simulink model "umpc_wl_qp_beckymod2"  (R2017a)
settings: Solver=FixedStepDiscrete  StartTime=0.0  StopTime=20  FixedStep=0.0002  RelTol=1e-3  EnableMultiTasking=on
values from neighbouring files (symbols this model uses):
  f_fin = f    (= 160)    [target_driver_setup.m]
  f_int = f    (= 160)    [target_driver_setup.m]
  kquad = [4e1, 1e-4, 4e-5, 153, 1e0]    [target_driver_setup.m]
  lpfParams = [0.2, 0.5, 1e-1, 1e1]    [target_driver_setup.m]
  phase = 0.0    (= 0)    [target_driver_setup.m]
  pos0 = [0.05,-0.02,0.08]    [target_driver_setup.m]
  running_time = 0.0+T+0.0    (= 2)    [target_driver_setup.m]
  start_delay = 0.0    (= 0)    [target_driver_setup.m]
  T = 2    [target_driver_setup.m]
  trajAmp = 0.07    [target_driver_setup.m]
  trajFreq = 0.5    [target_driver_setup.m]
  wmpc = single([3e2, 5e1, 1e-4, 2e-4, 1e0, 1e0, 1e-1, 1e0])    [target_driver_setup.m]
undefined symbols (not defined in the file or in its folder): Com1, DiscIntNeverNeededParam, none
libraries: simulink x9, xpcnilib x2, xpcseriallib x2, xpcutilitieslib x1

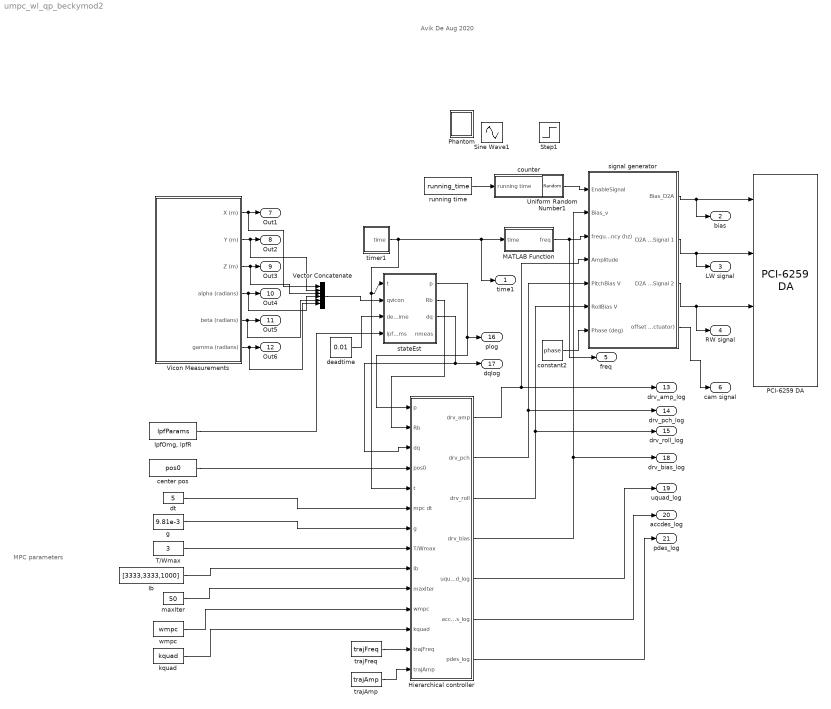
== system umpc_wl_qp_beckymod2 ==
  note: Avik De
      | Aug 2020
  note: MPC parameters
  Hierarchical controller : Subsystem
  Ib : Constant  Value=[3333,3333,1000]  OutDataTypeStr=single  SampleTime=-1
  MATLAB Function : MATLAB Function  TreatAsAtomicUnit=on
  PCI-6259 DA : xpcnilib/D//A/M Series/PCI-6259 DA  channel=[1:4]  range=[10,5, 10, 10]  reset=[1 1 1 1]  initValue=[0 0 0 0]  sampletime=-1  slot=-1
  Phantom : Subsystem
  T/Wmax : Constant  Value=3  OutDataTypeStr=single  SampleTime=-1
  Vector Concatenate : Concatenate  NumInputs=6
  Vicon Measurements : Subsystem
  center pos : Constant  Value=pos0  OutDataTypeStr=single  SampleTime=-1
  constant2 : Constant  Value=phase
  counter : Subsystem
  deadtime : Constant  Value=0.01
  dt : Constant  Value=5  OutDataTypeStr=single  SampleTime=-1
  g : Constant  Value=9.81e-3  OutDataTypeStr=single  SampleTime=-1
  kquad : Constant  Value=kquad  VectorParams1D=off  OutDataTypeStr=single  SampleTime=-1
  "lpfOmg, lpfR" : Constant  Value=lpfParams  VectorParams1D=off  OutDataTypeStr=double  SampleTime=-1
  maxIter : Constant  Value=50  OutDataTypeStr=int32  SampleTime=-1
  running time : Constant  Value=running_time  SampleTime=-1
  signal generator : Subsystem
  stateEst : MATLAB Function  TreatAsAtomicUnit=on
  timer1 : Subsystem
  trajAmp : Constant  Value=trajAmp  OutDataTypeStr=single  SampleTime=-1
  trajFreq : Constant  Value=trajFreq  OutDataTypeStr=single  SampleTime=-1
  wmpc : Constant  Value=wmpc  VectorParams1D=off  OutDataTypeStr=single  SampleTime=-1
  time1 : Outport
  bias : Outport  Port=2
  LW signal : Outport  Port=3
  RW signal : Outport  Port=4
  freq : Outport  Port=5
  cam signal : Outport  Port=6
  Out1 : Outport  Port=7
  Out2 : Outport  Port=8
  Out3 : Outport  Port=9
  Out4 : Outport  Port=10
  Out5 : Outport  Port=11
  Out6 : Outport  Port=12
  drv_amp_log : Outport  Port=13
  drv_pch_log : Outport  Port=14
  drv_roll_log : Outport  Port=15
  plog : Outport  Port=16
  dqlog : Outport  Port=17
  drv_bias_log : Outport  Port=18
  uquad_log : Outport  Port=19
  accdes_log : Outport  Port=20
  pdes_log : Outport  Port=21
  Sine Wave1 : Sin  IOType=siggen  SampleTime=0
  Step1 : Step  IOType=siggen  SampleTime=0
  Uniform Random Number1 : UniformRandomNumber  IOType=siggen  SampleTime=0
  wires:
  running time/1 -> counter/1(running time)
  signal generator/1(Bias_D2A) -> bias/1, PCI-6259 DA/1
  signal generator/2(D2A DriveSignal 1) -> LW signal/1, PCI-6259 DA/2
  signal generator/3(D2A DriveSignal 2) -> RW signal/1, PCI-6259 DA/3
  timer1/1(time) -> Hierarchical controller/5(t), stateEst/1(t), time1/1, MATLAB Function/1(time)
  counter/1(enable) -> signal generator/1(EnableSignal)
  MATLAB Function/1(freq) -> signal generator/3(frequency (hz)), freq/1
  signal generator/4(offset (for sylvain's actuator)) -> cam signal/1
  constant2/1 -> signal generator/7(Phase (deg))
  Vicon Measurements/1(X (m)) -> Vector Concatenate/1, Out1/1
  Vicon Measurements/6(gamma (radians)) -> Vector Concatenate/6, Out6/1
  Vicon Measurements/3(Z (m)) -> Vector Concatenate/3, Out3/1
  Vicon Measurements/2(Y (m)) -> Vector Concatenate/2, Out2/1
  Vicon Measurements/5(beta (radians)) -> Vector Concatenate/5, Out5/1
  Vicon Measurements/4(alpha (radians)) -> Vector Concatenate/4, Out4/1
  Hierarchical controller/1(drv_amp) -> drv_amp_log/1, signal generator/4(Amplitude)
  Hierarchical controller/3(drv_roll) -> signal generator/6(RollBias V), drv_roll_log/1
  Hierarchical controller/2(drv_pch) -> signal generator/5(PitchBias V), drv_pch_log/1
  stateEst/1(p) -> Hierarchical controller/1(p), plog/1
  stateEst/2(Rb) -> Hierarchical controller/2(Rb)
  stateEst/3(dq) -> dqlog/1, Hierarchical controller/3(dq)
  Vector Concatenate/1 -> stateEst/2(qvicon)
  Hierarchical controller/4(drv_bias) -> signal generator/2(Bias_v), drv_bias_log/1
  center pos/1 -> Hierarchical controller/4(pos0)
  dt/1 -> Hierarchical controller/6(mpc dt)
  g/1 -> Hierarchical controller/7(g)
  T/Wmax/1 -> Hierarchical controller/8(T/Wmax)
  wmpc/1 -> Hierarchical controller/11(wmpc)
  maxIter/1 -> Hierarchical controller/10(maxIter)
  Ib/1 -> Hierarchical controller/9(Ib)
  Hierarchical controller/5(uquad_log) -> uquad_log/1
  Hierarchical controller/6(accdes_log) -> accdes_log/1
  deadtime/1 -> stateEst/3(deadtime)
  kquad/1 -> Hierarchical controller/12(kquad)
  "lpfOmg, lpfR"/1 -> stateEst/4(lpfParams)
  Hierarchical controller/7(pdes_log) -> pdes_log/1
  trajFreq/1 -> Hierarchical controller/13(trajFreq)
  trajAmp/1 -> Hierarchical controller/14(trajAmp)

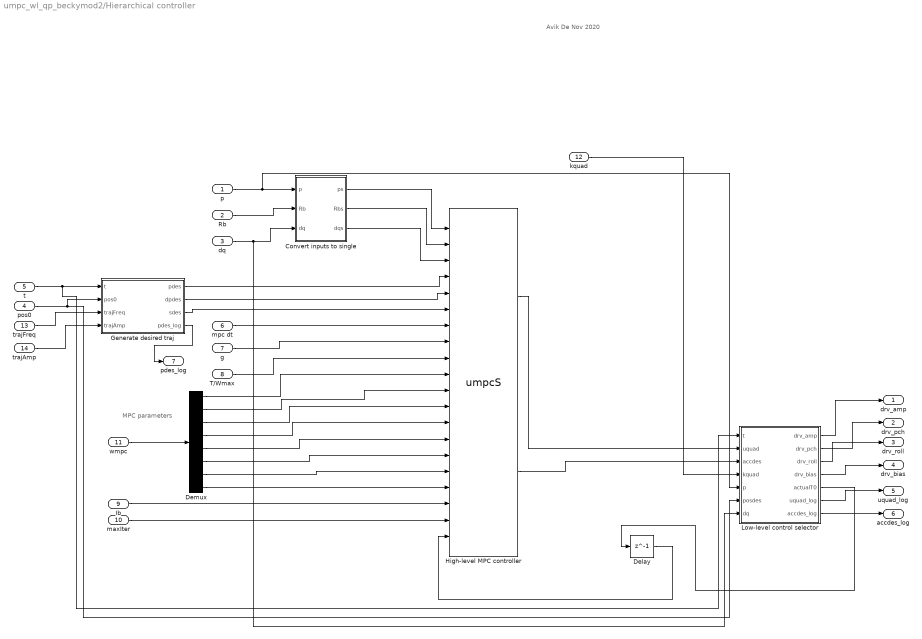
== system umpc_wl_qp_beckymod2/Hierarchical controller ==
  note: Avik De
      | Nov 2020
  note: MPC parameters
  p : Inport
  Rb : Inport  Port=2
  dq : Inport  Port=3
  pos0 : Inport  Port=4
  t : Inport  Port=5
  mpc dt : Inport  Port=6
  g : Inport  Port=7
  T/Wmax : Inport  Port=8
  Ib : Inport  Port=9
  maxIter : Inport  Port=10
  wmpc : Inport  Port=11
  kquad : Inport  Port=12
  trajFreq : Inport  Port=13
  trajAmp : Inport  Port=14
  Convert inputs to single : MATLAB Function  TreatAsAtomicUnit=on
  Delay : Delay  DelayLength=1  InitialCondition=0
  Demux : Demux  Outputs=8
  Generate desired traj : MATLAB Function  TreatAsAtomicUnit=on
  High-level MPC controller : S-Function  FunctionName=umpcS  Parameters=SampleTime  SFunctionDeploymentMode=off  EnableBusSupport=off  mask(Legacy Function){SFunctionSpec=void umpcS(single y1[3], single y2[6], single u1[3], single u2[3][3], single u3[6], single u4[3], single u5[3], single u6[3], single u7, single u8, single u9, single u10, single u11, single u12, single u13, single u14, single u15, single u16, single u17, single u18[3], int32 u19, single u20), SampleTime=-1, ShowSpec=off}
      mask prompts: SampleTime "Sample time (-1 for inherited):"; ShowSpec "Display function specification"
      mask help: This block allows you to call the legacy functions specified by the following Legacy Code Tool definition: def.SFunctionName = 'umpcS'; def.OutputFcnSpec = 'void umpcS(single y1[3], single y2[6], single u1[3], single u2[3][3], single u3[6], single u4[3], single u5[3], single u6[3], single u7, single u8, single u9, single u10, single u11, single u12, single u13, single u14, single u15, single u16, single u17, single u18[3], int32 u19, single u20)'; def.HeaderFiles = {'uprightmpc2.h'}; def.SourceFiles = {'uprightmpc2.c', 'eigenc.c', 'auxil.c', 'error.c', 'kkt.c', 'lin_alg.c', 'osqp.c', 'proj.c',
  Low-level control selector : MATLAB Function  TreatAsAtomicUnit=on
  drv_amp : Outport
  drv_pch : Outport  Port=2
  drv_roll : Outport  Port=3
  drv_bias : Outport  Port=4
  uquad_log : Outport  Port=5
  accdes_log : Outport  Port=6
  pdes_log : Outport  Port=7  OutDataTypeStr=double
  wires:
  Low-level control selector/2(drv_pch) -> drv_pch/1
  Low-level control selector/3(drv_roll) -> drv_roll/1
  Low-level control selector/4(drv_bias) -> drv_bias/1
  Low-level control selector/1(drv_amp) -> drv_amp/1
  pos0/1 -> Low-level control selector/6(posdes), Generate desired traj/2(pos0)
  mpc dt/1 -> High-level MPC controller/7
  g/1 -> High-level MPC controller/8
  T/Wmax/1 -> High-level MPC controller/9
  Demux/1 -> High-level MPC controller/10
  Demux/2 -> High-level MPC controller/11
  Demux/3 -> High-level MPC controller/12
  Demux/4 -> High-level MPC controller/13
  Demux/5 -> High-level MPC controller/14
  Demux/6 -> High-level MPC controller/15
  Demux/7 -> High-level MPC controller/16
  Demux/8 -> High-level MPC controller/17
  Ib/1 -> High-level MPC controller/18
  maxIter/1 -> High-level MPC controller/19
  High-level MPC controller/1 -> Low-level control selector/2(uquad)
  t/1 -> Low-level control selector/1(t), Generate desired traj/1(t)
  Generate desired traj/1(pdes) -> High-level MPC controller/4
  Generate desired traj/2(dpdes) -> High-level MPC controller/5
  Convert inputs to single/1(ps) -> High-level MPC controller/1
  Convert inputs to single/2(Rbs) -> High-level MPC controller/2
  Convert inputs to single/3(dqs) -> High-level MPC controller/3
  p/1 -> Low-level control selector/5(p), Convert inputs to single/1(p)
  Rb/1 -> Convert inputs to single/2(Rb)
  dq/1 -> Low-level control selector/7(dq), Convert inputs to single/3(dq)
  High-level MPC controller/2 -> Low-level control selector/3(accdes)
  Generate desired traj/3(sdes) -> High-level MPC controller/6
  Low-level control selector/6(uquad_log) -> uquad_log/1
  Low-level control selector/7(accdes_log) -> accdes_log/1
  Low-level control selector/5(actualT0) -> Delay/1
  Delay/1 -> High-level MPC controller/20
  wmpc/1 -> Demux/1
  kquad/1 -> Low-level control selector/4(kquad)
  trajFreq/1 -> Generate desired traj/3(trajFreq)
  trajAmp/1 -> Generate desired traj/4(trajAmp)
  Generate desired traj/4(pdes_log) -> pdes_log/1

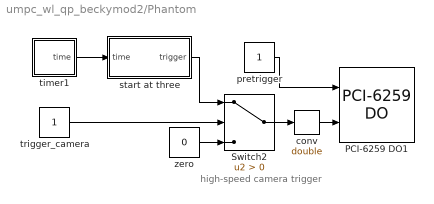
== system umpc_wl_qp_beckymod2/Phantom ==
  note: high-speed camera trigger
  PCI-6259 DO1 : xpcnilib/Digital Output/M Series/PCI-6259 DO  channel=[1 2]  reset=[0 0]  initValue=[0 0]  sampletime=0.0002  slot=-1
  Switch2 : Switch  Criteria=u2 > Threshold
  conv : DataTypeConversion  OutDataTypeStr=double
  pretrigger : Constant
  start at three : MATLAB Function  TreatAsAtomicUnit=on
  timer1 : Subsystem
  trigger_camera : Constant
  zero : Constant  Value=0
  wires:
  timer1/1(time) -> start at three/1(time)
  start at three/1(trigger) -> Switch2/1
  Switch2/1 -> conv/1
  zero/1 -> Switch2/3
  trigger_camera/1 -> Switch2/2
  conv/1 -> PCI-6259 DO1/2
  pretrigger/1 -> PCI-6259 DO1/1

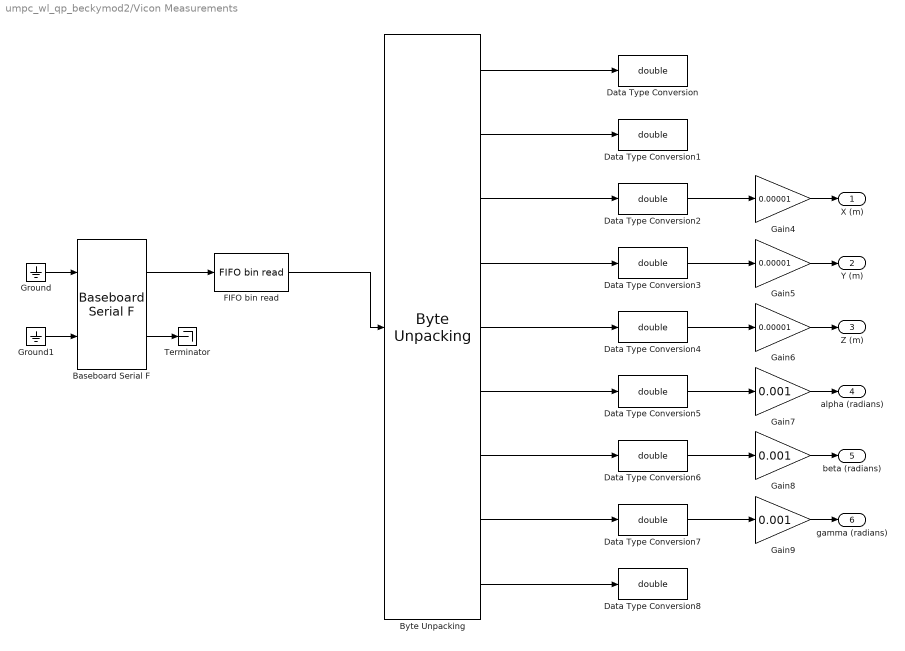
== system umpc_wl_qp_beckymod2/Vicon Measurements ==
  Baseboard Serial F : xpcseriallib/Mainboard/Baseboard Serial F  group=FIFO Setup  port=1  irqnum=4  saddr1=0x3f8  saddr2=0x3e8  config=Com1/none  baud1=115200  parity1=None  ndata1=8  nstop1=1  fifomode1=16 deep  rlevel1=half full  automode1=on  xmtfifosize1=1024  xmtdatatype1=8 bit int null terminated  rcvfifosize1=1024  baud2=115200  parity2=None  ndata2=8  nstop2=1  fifomode2=16 deep  rlevel2=half full  automode2=off  xmtfifosize2=1024  xmtdatatype2=8 bit uint null terminated  rcvfifosize2=1024
  "Byte Unpacking " : xpcutilitieslib/Byte Unpacking   MaskUnpackedDataTypes={'uint8','int16','int16','int16','int16','int16','int16','int16','uint8'}  MaskUnpackedDataSizes={[1] [1] [1] [1] [1] [1] [1] [1] [1]}  MaskAlignment=1
  Data Type Conversion{,1..8} (9 alike) : DataTypeConversion  OutDataTypeStr=double
  "FIFO bin read " : xpcseriallib/FIFO bin read   header=[128,127,127]  lengths=[15]  hold=Hold last output if no new data  enable=off  maxsize=15  outputtype=8 bit uint null terminated  sampletime=0.0002
  Gain4 : Gain  Gain=0.00001
  Gain5 : Gain  Gain=0.00001
  Gain6 : Gain  Gain=0.00001
  Gain7 : Gain  Gain=0.001
  Gain8 : Gain  Gain=0.001
  Gain9 : Gain  Gain=0.001
  Ground : Ground
  Ground1 : Ground
  Terminator : Terminator
  X (m) : Outport
  Y (m) : Outport  Port=2
  Z (m) : Outport  Port=3
  alpha (radians) : Outport  Port=4
  beta (radians) : Outport  Port=5
  gamma (radians) : Outport  Port=6
  wires:
  Baseboard Serial F/1 -> "FIFO bin read "/1
  Baseboard Serial F/2 -> Terminator/1
  Ground1/1 -> Baseboard Serial F/2
  Ground/1 -> Baseboard Serial F/1
  "Byte Unpacking "/1 -> Data Type Conversion/1
  "Byte Unpacking "/2 -> Data Type Conversion1/1
  "Byte Unpacking "/3 -> Data Type Conversion2/1
  "Byte Unpacking "/4 -> Data Type Conversion3/1
  "FIFO bin read "/1 -> "Byte Unpacking "/1
  "Byte Unpacking "/8 -> Data Type Conversion7/1
  "Byte Unpacking "/7 -> Data Type Conversion6/1
  "Byte Unpacking "/5 -> Data Type Conversion4/1
  "Byte Unpacking "/6 -> Data Type Conversion5/1
  Data Type Conversion3/1 -> Gain5/1
  Data Type Conversion4/1 -> Gain6/1
  Data Type Conversion5/1 -> Gain7/1
  Data Type Conversion6/1 -> Gain8/1
  Data Type Conversion7/1 -> Gain9/1
  "Byte Unpacking "/9 -> Data Type Conversion8/1
  Gain4/1 -> X (m)/1
  Data Type Conversion2/1 -> Gain4/1
  Gain5/1 -> Y (m)/1
  Gain6/1 -> Z (m)/1
  Gain7/1 -> alpha (radians)/1
  Gain8/1 -> beta (radians)/1
  Gain9/1 -> gamma (radians)/1

== system umpc_wl_qp_beckymod2/counter ==
  running time : Inport
  Add : Sum  Inputs=+-
  Compare To Zero : simulink/Logic and Bit Operations/Compare To Zero  relop=<  OutDataTypeStr=uint8  ZeroCross=off
  Product2 : Product  RndMeth=Zero
  SaturatingRamp : DiscreteIntegrator  gainval=1  SampleTime=-1  UpperSaturationLimit=1  LowerSaturationLimit=0  ICPrevOutput=DiscIntNeverNeededParam  ICPrevScaledInput=DiscIntNeverNeededParam
  constant : Constant
  start delay compare : simulink/Logic and Bit Operations/Compare To Constant  relop=>  const=start_delay  OutDataTypeStr=uint8
  enable : Outport
  wires:
  SaturatingRamp/1 -> Add/1, start delay compare/1
  running time/1 -> Add/2
  Add/1 -> Compare To Zero/1
  start delay compare/1 -> Product2/1
  Compare To Zero/1 -> Product2/2
  Product2/1 -> enable/1
  constant/1 -> SaturatingRamp/1

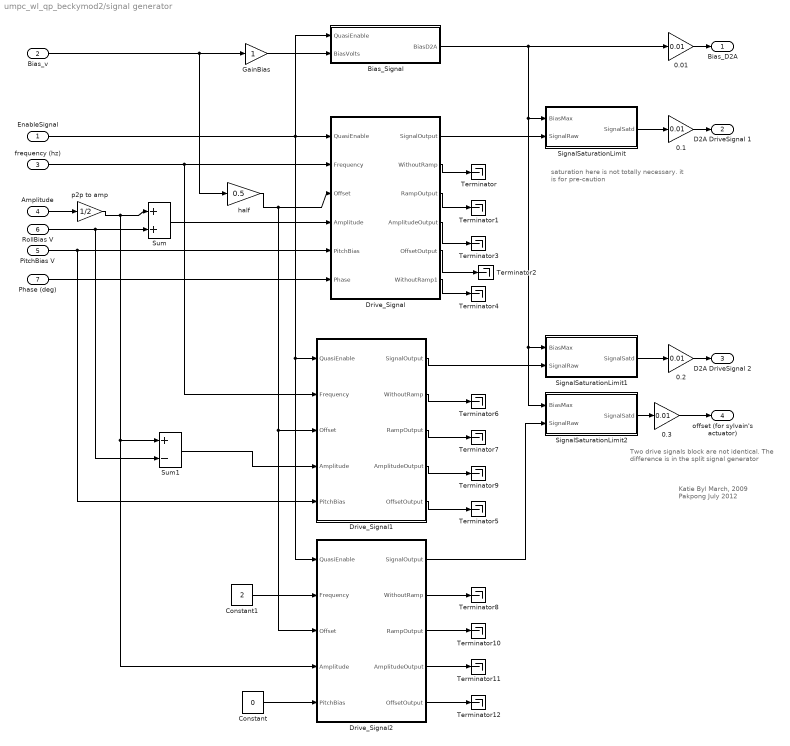
== system umpc_wl_qp_beckymod2/signal generator ==
  note: Katie Byl
      | March, 2009
      |
      | Pakpong
      | July 2012
  note: Two drive signals block are not identical.
      | The difference is in the split signal generator
  note: saturation here is not totally necessary.
      | it is for pre-caution
  EnableSignal : Inport
  Bias_v : Inport  Port=2
  frequency (hz) : Inport  Port=3
  Amplitude : Inport  Port=4
  PitchBias V : Inport  Port=5
  RollBias V : Inport  Port=6
  Phase (deg) : Inport  Port=7
  0.01 : Gain  Gain=0.01
  0.1 : Gain  Gain=0.01
  0.2 : Gain  Gain=0.01
  0.3 : Gain  Gain=0.01
  Bias_Signal : Subsystem
  Constant : Constant  Value=0
  Constant1 : Constant  Value=2
  Drive_Signal : Subsystem
  Drive_Signal1 : Subsystem
  Drive_Signal2 : Subsystem
  GainBias : Gain
  SignalSaturationLimit : Subsystem
  SignalSaturationLimit1 : Subsystem
  SignalSaturationLimit2 : Subsystem
  Sum : Sum
  Sum1 : Sum  Inputs=+-
  Terminator{,1..12} (13 alike) : Terminator
  half : Gain  Gain=0.5
  p2p to amp : Gain  Gain=1/2
  Bias_D2A : Outport
  D2A DriveSignal 1 : Outport  Port=2
  D2A DriveSignal 2 : Outport  Port=3
  offset (for sylvain's actuator) : Outport  Port=4
  wires:
  Bias_Signal/1(BiasD2A) -> SignalSaturationLimit1/1(BiasMax), SignalSaturationLimit2/1(BiasMax), SignalSaturationLimit/1(BiasMax), 0.01/1
  half/1 -> Drive_Signal/3(Offset), Drive_Signal1/3(Offset), Drive_Signal2/3(Offset)
  Bias_v/1 -> GainBias/1, half/1
  EnableSignal/1 -> Drive_Signal/1(QuasiEnable), Bias_Signal/1(QuasiEnable), Drive_Signal1/1(QuasiEnable), Drive_Signal2/1(QuasiEnable)
  frequency (hz)/1 -> Drive_Signal1/2(Frequency), Drive_Signal/2(Frequency)
  Drive_Signal/2(WithoutRamp) -> Terminator/1
  Drive_Signal/3(RampOutput) -> Terminator1/1
  Drive_Signal/5(OffsetOutput) -> Terminator2/1
  SignalSaturationLimit/1(SignalSatd) -> 0.1/1
  GainBias/1 -> Bias_Signal/2(BiasVolts)
  PitchBias V/1 -> Drive_Signal/5(PitchBias), Drive_Signal1/5(PitchBias)
  Sum/1 -> Drive_Signal/4(Amplitude)
  RollBias V/1 -> Sum/2, Sum1/2
  SignalSaturationLimit1/1(SignalSatd) -> 0.2/1
  Drive_Signal1/5(OffsetOutput) -> Terminator5/1
  Amplitude/1 -> p2p to amp/1
  p2p to amp/1 -> Sum/1, Sum1/1, Drive_Signal2/4(Amplitude)
  Drive_Signal/4(AmplitudeOutput) -> Terminator3/1
  Drive_Signal1/2(WithoutRamp) -> Terminator6/1
  Drive_Signal1/3(RampOutput) -> Terminator7/1
  Drive_Signal1/4(AmplitudeOutput) -> Terminator9/1
  0.01/1 -> Bias_D2A/1
  0.1/1 -> D2A DriveSignal 1/1
  0.2/1 -> D2A DriveSignal 2/1
  Sum1/1 -> Drive_Signal1/4(Amplitude)
  0.3/1 -> offset (for sylvain's actuator)/1
  SignalSaturationLimit2/1(SignalSatd) -> 0.3/1
  Drive_Signal1/1(SignalOutput) -> SignalSaturationLimit1/2(SignalRaw)
  Drive_Signal/1(SignalOutput) -> SignalSaturationLimit/2(SignalRaw)
  Phase (deg)/1 -> Drive_Signal/6(Phase)
  Drive_Signal/6(WithoutRamp1) -> Terminator4/1
  Drive_Signal2/5(OffsetOutput) -> Terminator12/1
  Drive_Signal2/4(AmplitudeOutput) -> Terminator11/1
  Drive_Signal2/3(RampOutput) -> Terminator10/1
  Drive_Signal2/2(WithoutRamp) -> Terminator8/1
  Drive_Signal2/1(SignalOutput) -> SignalSaturationLimit2/2(SignalRaw)
  Constant/1 -> Drive_Signal2/5(PitchBias)
  Constant1/1 -> Drive_Signal2/2(Frequency)

== system umpc_wl_qp_beckymod2/timer1 ==
  SaturatingRamp : DiscreteIntegrator  gainval=1  SampleTime=-1  UpperSaturationLimit=1  LowerSaturationLimit=0  ICPrevOutput=DiscIntNeverNeededParam  ICPrevScaledInput=DiscIntNeverNeededParam
  constant : Constant
  time : Outport
  wires:
  SaturatingRamp/1 -> time/1
  constant/1 -> SaturatingRamp/1

== system umpc_wl_qp_beckymod2/Phantom/timer1 ==
  SaturatingRamp : DiscreteIntegrator  gainval=1  SampleTime=-1  UpperSaturationLimit=1  LowerSaturationLimit=0  ICPrevOutput=DiscIntNeverNeededParam  ICPrevScaledInput=DiscIntNeverNeededParam
  constant : Constant
  time : Outport
  wires:
  SaturatingRamp/1 -> time/1
  constant/1 -> SaturatingRamp/1

== system umpc_wl_qp_beckymod2/signal generator/Bias_Signal ==
  note: time constant = 0.002sec
  QuasiEnable : Inport
  BiasVolts : Inport  Port=2
  AveragedBias : Subsystem
  PreGain : Gain
  Product : Product  RndMeth=Zero
  SIgnalForRamp_binary : Subsystem
  SaturatingRamp : DiscreteIntegrator  gainval=10  SampleTime=-1  LimitOutput=on  UpperSaturationLimit=1  LowerSaturationLimit=0  ICPrevOutput=DiscIntNeverNeededParam  ICPrevScaledInput=DiscIntNeverNeededParam
  BiasD2A : Outport
  wires:
  PreGain/1 -> BiasD2A/1
  BiasVolts/1 -> AveragedBias/1(In1)
  QuasiEnable/1 -> SIgnalForRamp_binary/1(In1)
  SIgnalForRamp_binary/1(Out1) -> SaturatingRamp/1
  SaturatingRamp/1 -> Product/1
  AveragedBias/1(Out1) -> Product/2
  Product/1 -> PreGain/1

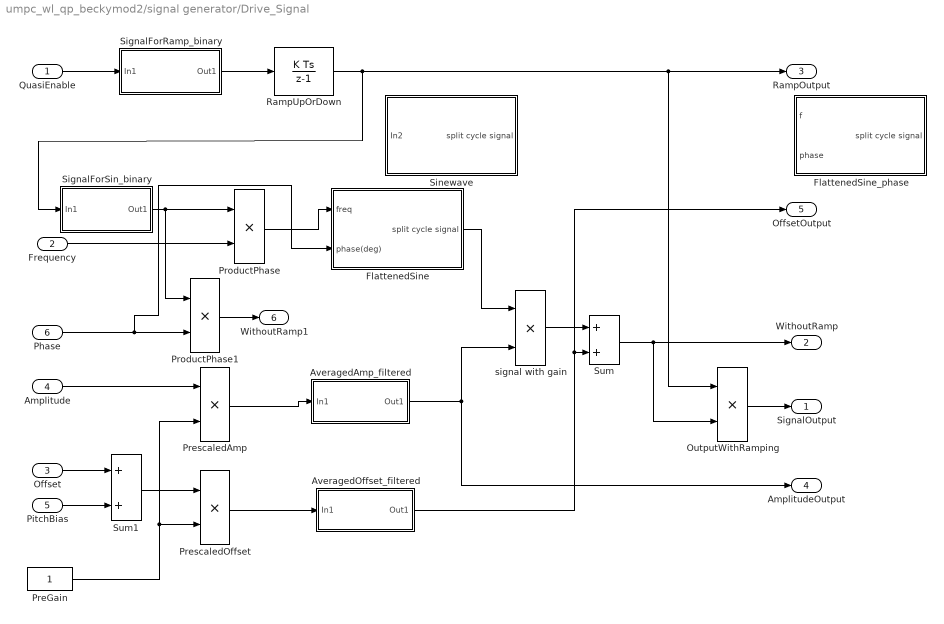
== system umpc_wl_qp_beckymod2/signal generator/Drive_Signal ==
  QuasiEnable : Inport
  Frequency : Inport  Port=2
  Offset : Inport  Port=3
  Amplitude : Inport  Port=4
  PitchBias : Inport  Port=5
  Phase : Inport  Port=6
  AveragedAmp_filtered : Subsystem
  AveragedOffset_filtered : Subsystem
  FlattenedSine : Subsystem
  FlattenedSine_phase : Subsystem
  OutputWithRamping : Product  RndMeth=Zero
  PreGain : Constant
  PrescaledAmp : Product  RndMeth=Zero
  PrescaledOffset : Product  RndMeth=Zero
  ProductPhase : Product  RndMeth=Zero
  ProductPhase1 : Product  RndMeth=Zero
  RampUpOrDown : DiscreteIntegrator  gainval=10  SampleTime=-1  LimitOutput=on  UpperSaturationLimit=1  LowerSaturationLimit=0  ICPrevOutput=DiscIntNeverNeededParam  ICPrevScaledInput=DiscIntNeverNeededParam
  SignalForRamp_binary : Subsystem
  SignalForSin_binary : Subsystem
  Sinewave : Subsystem
  Sum : Sum
  Sum1 : Sum
  signal with gain : Product  RndMeth=Zero
  SignalOutput : Outport
  WithoutRamp : Outport  Port=2
  RampOutput : Outport  Port=3
  AmplitudeOutput : Outport  Port=4
  OffsetOutput : Outport  Port=5
  WithoutRamp1 : Outport  Port=6
  wires:
  PrescaledAmp/1 -> AveragedAmp_filtered/1(In1)
  Sum/1 -> OutputWithRamping/2, WithoutRamp/1
  RampUpOrDown/1 -> RampOutput/1, OutputWithRamping/1, SignalForSin_binary/1(In1)
  QuasiEnable/1 -> SignalForRamp_binary/1(In1)
  SignalForRamp_binary/1(Out1) -> RampUpOrDown/1
  Amplitude/1 -> PrescaledAmp/1
  signal with gain/1 -> Sum/1
  Frequency/1 -> ProductPhase/2
  SignalForSin_binary/1(Out1) -> ProductPhase/1, ProductPhase1/1
  AveragedOffset_filtered/1(Out1) -> Sum/2, OffsetOutput/1
  PrescaledOffset/1 -> AveragedOffset_filtered/1(In1)
  PreGain/1 -> PrescaledAmp/2, PrescaledOffset/2
  OutputWithRamping/1 -> SignalOutput/1
  AveragedAmp_filtered/1(Out1) -> signal with gain/2, AmplitudeOutput/1
  Sum1/1 -> PrescaledOffset/1
  Offset/1 -> Sum1/1
  PitchBias/1 -> Sum1/2
  Phase/1 -> FlattenedSine/2(phase(deg)), ProductPhase1/2
  ProductPhase1/1 -> WithoutRamp1/1
  ProductPhase/1 -> FlattenedSine/1(freq)
  FlattenedSine/1(split cycle signal) -> signal with gain/1

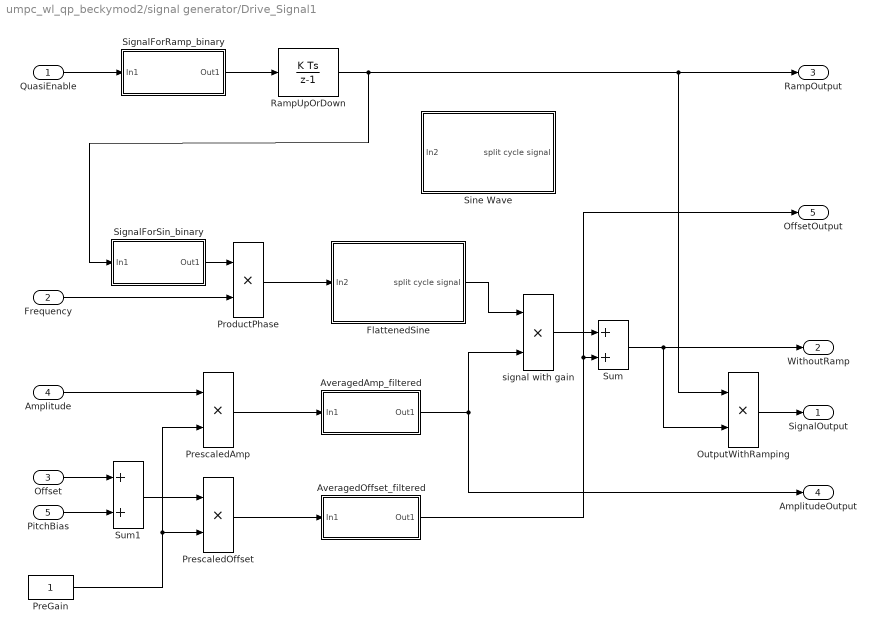
== system umpc_wl_qp_beckymod2/signal generator/Drive_Signal1 ==
  QuasiEnable : Inport
  Frequency : Inport  Port=2
  Offset : Inport  Port=3
  Amplitude : Inport  Port=4
  PitchBias : Inport  Port=5
  AveragedAmp_filtered : Subsystem
  AveragedOffset_filtered : Subsystem
  FlattenedSine : Subsystem
  OutputWithRamping : Product  RndMeth=Zero
  PreGain : Constant
  PrescaledAmp : Product  RndMeth=Zero
  PrescaledOffset : Product  RndMeth=Zero
  ProductPhase : Product  RndMeth=Zero
  RampUpOrDown : DiscreteIntegrator  gainval=10  SampleTime=-1  LimitOutput=on  UpperSaturationLimit=1  LowerSaturationLimit=0  ICPrevOutput=DiscIntNeverNeededParam  ICPrevScaledInput=DiscIntNeverNeededParam
  SignalForRamp_binary : Subsystem
  SignalForSin_binary : Subsystem
  Sine Wave : Subsystem
  Sum : Sum
  Sum1 : Sum
  signal with gain : Product  RndMeth=Zero
  SignalOutput : Outport
  WithoutRamp : Outport  Port=2
  RampOutput : Outport  Port=3
  AmplitudeOutput : Outport  Port=4
  OffsetOutput : Outport  Port=5
  wires:
  PrescaledAmp/1 -> AveragedAmp_filtered/1(In1)
  Sum/1 -> OutputWithRamping/2, WithoutRamp/1
  RampUpOrDown/1 -> RampOutput/1, OutputWithRamping/1, SignalForSin_binary/1(In1)
  QuasiEnable/1 -> SignalForRamp_binary/1(In1)
  SignalForRamp_binary/1(Out1) -> RampUpOrDown/1
  signal with gain/1 -> Sum/1
  Frequency/1 -> ProductPhase/2
  SignalForSin_binary/1(Out1) -> ProductPhase/1
  AveragedOffset_filtered/1(Out1) -> Sum/2, OffsetOutput/1
  PrescaledOffset/1 -> AveragedOffset_filtered/1(In1)
  PreGain/1 -> PrescaledAmp/2, PrescaledOffset/2
  OutputWithRamping/1 -> SignalOutput/1
  AveragedAmp_filtered/1(Out1) -> signal with gain/2, AmplitudeOutput/1
  Sum1/1 -> PrescaledOffset/1
  Offset/1 -> Sum1/1
  PitchBias/1 -> Sum1/2
  Amplitude/1 -> PrescaledAmp/1
  FlattenedSine/1(split cycle signal) -> signal with gain/1
  ProductPhase/1 -> FlattenedSine/1(In2)

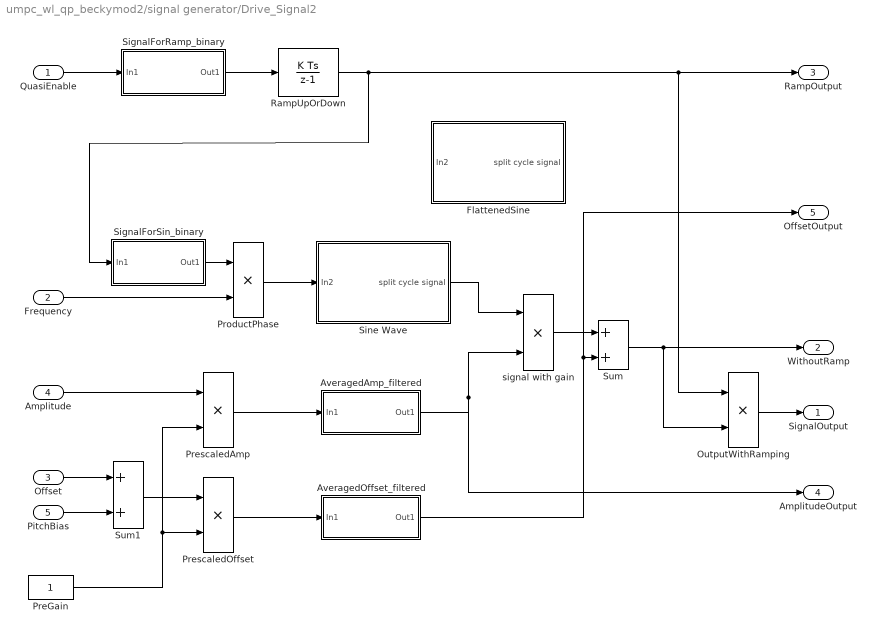
== system umpc_wl_qp_beckymod2/signal generator/Drive_Signal2 ==
  QuasiEnable : Inport
  Frequency : Inport  Port=2
  Offset : Inport  Port=3
  Amplitude : Inport  Port=4
  PitchBias : Inport  Port=5
  AveragedAmp_filtered : Subsystem
  AveragedOffset_filtered : Subsystem
  FlattenedSine : Subsystem
  OutputWithRamping : Product  RndMeth=Zero
  PreGain : Constant
  PrescaledAmp : Product  RndMeth=Zero
  PrescaledOffset : Product  RndMeth=Zero
  ProductPhase : Product  RndMeth=Zero
  RampUpOrDown : DiscreteIntegrator  gainval=10  SampleTime=-1  LimitOutput=on  UpperSaturationLimit=1  LowerSaturationLimit=0  ICPrevOutput=DiscIntNeverNeededParam  ICPrevScaledInput=DiscIntNeverNeededParam
  SignalForRamp_binary : Subsystem
  SignalForSin_binary : Subsystem
  Sine Wave : Subsystem
  Sum : Sum
  Sum1 : Sum
  signal with gain : Product  RndMeth=Zero
  SignalOutput : Outport
  WithoutRamp : Outport  Port=2
  RampOutput : Outport  Port=3
  AmplitudeOutput : Outport  Port=4
  OffsetOutput : Outport  Port=5
  wires:
  PrescaledAmp/1 -> AveragedAmp_filtered/1(In1)
  Sum/1 -> OutputWithRamping/2, WithoutRamp/1
  RampUpOrDown/1 -> RampOutput/1, OutputWithRamping/1, SignalForSin_binary/1(In1)
  QuasiEnable/1 -> SignalForRamp_binary/1(In1)
  SignalForRamp_binary/1(Out1) -> RampUpOrDown/1
  signal with gain/1 -> Sum/1
  Frequency/1 -> ProductPhase/2
  SignalForSin_binary/1(Out1) -> ProductPhase/1
  AveragedOffset_filtered/1(Out1) -> Sum/2, OffsetOutput/1
  PrescaledOffset/1 -> AveragedOffset_filtered/1(In1)
  PreGain/1 -> PrescaledAmp/2, PrescaledOffset/2
  OutputWithRamping/1 -> SignalOutput/1
  AveragedAmp_filtered/1(Out1) -> signal with gain/2, AmplitudeOutput/1
  Sum1/1 -> PrescaledOffset/1
  Offset/1 -> Sum1/1
  PitchBias/1 -> Sum1/2
  Amplitude/1 -> PrescaledAmp/1
  ProductPhase/1 -> Sine Wave/1(In2)
  Sine Wave/1(split cycle signal) -> signal with gain/1

== system umpc_wl_qp_beckymod2/signal generator/SignalSaturationLimit ==
  BiasMax : Inport
  SignalRaw : Inport  Port=2
  GainBias : Gain
  MaxOf : MinMax  Function=max  Inputs=2
  MinOf : MinMax  Inputs=2
  ground : Constant
  SignalSatd : Outport
  wires:
  BiasMax/1 -> GainBias/1
  SignalRaw/1 -> MinOf/2
  MinOf/1 -> MaxOf/1
  MaxOf/1 -> SignalSatd/1
  GainBias/1 -> MinOf/1
  ground/1 -> MaxOf/2

== system umpc_wl_qp_beckymod2/signal generator/SignalSaturationLimit1 ==
  BiasMax : Inport
  SignalRaw : Inport  Port=2
  GainBias : Gain
  MaxOf : MinMax  Function=max  Inputs=2
  MinOf : MinMax  Inputs=2
  ground : Constant
  SignalSatd : Outport
  wires:
  BiasMax/1 -> GainBias/1
  SignalRaw/1 -> MinOf/2
  MinOf/1 -> MaxOf/1
  MaxOf/1 -> SignalSatd/1
  GainBias/1 -> MinOf/1
  ground/1 -> MaxOf/2

== system umpc_wl_qp_beckymod2/signal generator/SignalSaturationLimit2 ==
  BiasMax : Inport
  SignalRaw : Inport  Port=2
  GainBias : Gain
  MaxOf : MinMax  Function=max  Inputs=2
  MinOf : MinMax  Inputs=2
  ground : Constant
  SignalSatd : Outport
  wires:
  BiasMax/1 -> GainBias/1
  SignalRaw/1 -> MinOf/2
  MinOf/1 -> MaxOf/1
  MaxOf/1 -> SignalSatd/1
  GainBias/1 -> MinOf/1
  ground/1 -> MaxOf/2

== system umpc_wl_qp_beckymod2/signal generator/Bias_Signal/AveragedBias ==
  note: To avoid having signal "jump",
      | we want SMOOTH transitions
      | in frequency (i.e., a weighted sum
      | of current freq and freq some delta t ago)
  note: time constant = 0.002sec
  In1 : Inport
  Discrete Transfer Fcn : DiscreteTransferFcn  Numerator=[0.05]  Denominator=[1 -.95]
  Out1 : Outport
  wires:
  In1/1 -> Discrete Transfer Fcn/1
  Discrete Transfer Fcn/1 -> Out1/1

== system umpc_wl_qp_beckymod2/signal generator/Bias_Signal/SIgnalForRamp_binary ==
  note: Should output 1 or -1,
      | so signal ramps UP to 1
      | or DOWN to 0.
  In1 : Inport
  Add : Sum  Inputs=+-
  Compare To Zero : simulink/Logic and Bit Operations/Compare To Zero  relop=>  OutDataTypeStr=uint8  ZeroCross=off
  Constant : Constant
  Data Type Conversion : DataTypeConversion  OutDataTypeStr=double
  Gain : Gain  Gain=2
  Out1 : Outport
  wires:
  In1/1 -> Compare To Zero/1
  Compare To Zero/1 -> Data Type Conversion/1
  Gain/1 -> Add/1
  Constant/1 -> Add/2
  Add/1 -> Out1/1
  Data Type Conversion/1 -> Gain/1

== system umpc_wl_qp_beckymod2/signal generator/Drive_Signal/AveragedAmp_filtered ==
  note: To avoid having signal "jump",
      | we want SMOOTH transitions
      | in frequency (i.e., a weighted sum
      | of current freq and freq some delta t ago)
  note: time constant 0.002sec
      | for 10kHz samping
  In1 : Inport
  Discrete Transfer Fcn : DiscreteTransferFcn  Numerator=[0.05]  Denominator=[1 -.95]
  Out1 : Outport
  wires:
  In1/1 -> Discrete Transfer Fcn/1
  Discrete Transfer Fcn/1 -> Out1/1

== system umpc_wl_qp_beckymod2/signal generator/Drive_Signal/AveragedOffset_filtered ==
  note: To avoid having signal "jump",
      | we want SMOOTH transitions
      | in frequency (i.e., a weighted sum
      | of current freq and freq some delta t ago)
  note: c
  note: time constant 0.02sec
      | for 10kHz samping
  In1 : Inport
  Discrete Transfer Fcn : DiscreteTransferFcn  Numerator=[0.05]  Denominator=[1 -.95]
  Out1 : Outport
  wires:
  In1/1 -> Discrete Transfer Fcn/1
  Discrete Transfer Fcn/1 -> Out1/1

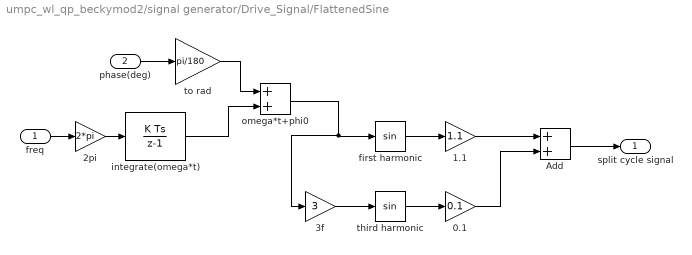
== system umpc_wl_qp_beckymod2/signal generator/Drive_Signal/FlattenedSine ==
  freq : Inport
  phase(deg) : Inport  Port=2
  0.1 : Gain  Gain=0.1
  1.1 : Gain  Gain=1.1
  2pi : Gain  Gain=2*pi
  3f : Gain  Gain=3
  Add : Sum
  first harmonic : Trigonometry  OutputSignalType=real
  integrate(omega*t) : DiscreteIntegrator  SampleTime=-1  ICPrevOutput=DiscIntNeverNeededParam  ICPrevScaledInput=DiscIntNeverNeededParam
  omega*t+phi0 : Sum
  third harmonic : Trigonometry  OutputSignalType=real
  to rad : Gain  Gain=pi/180
  split cycle signal : Outport
  wires:
  freq/1 -> 2pi/1
  2pi/1 -> integrate(omega*t)/1
  3f/1 -> third harmonic/1
  first harmonic/1 -> 1.1/1
  third harmonic/1 -> 0.1/1
  1.1/1 -> Add/1
  0.1/1 -> Add/2
  Add/1 -> split cycle signal/1
  integrate(omega*t)/1 -> omega*t+phi0/2
  omega*t+phi0/1 -> 3f/1, first harmonic/1
  phase(deg)/1 -> to rad/1
  to rad/1 -> omega*t+phi0/1

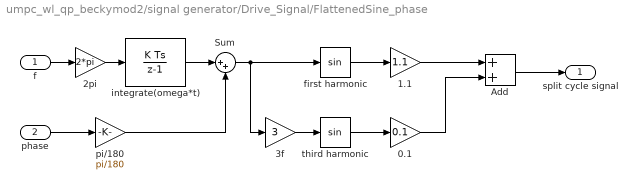
== system umpc_wl_qp_beckymod2/signal generator/Drive_Signal/FlattenedSine_phase ==
  f : Inport
  phase : Inport  Port=2
  0.1 : Gain  Gain=0.1
  1.1 : Gain  Gain=1.1
  2pi : Gain  Gain=2*pi
  3f : Gain  Gain=3
  Add : Sum
  Sum : Sum  Inputs=|++
  first harmonic : Trigonometry  OutputSignalType=real
  integrate(omega*t) : DiscreteIntegrator  SampleTime=-1  ICPrevOutput=DiscIntNeverNeededParam  ICPrevScaledInput=DiscIntNeverNeededParam
  pi/180 : Gain  Gain=pi/180
  third harmonic : Trigonometry  OutputSignalType=real
  split cycle signal : Outport
  wires:
  f/1 -> 2pi/1
  2pi/1 -> integrate(omega*t)/1
  3f/1 -> third harmonic/1
  first harmonic/1 -> 1.1/1
  third harmonic/1 -> 0.1/1
  1.1/1 -> Add/1
  0.1/1 -> Add/2
  Add/1 -> split cycle signal/1
  Sum/1 -> first harmonic/1, 3f/1
  pi/180/1 -> Sum/2
  integrate(omega*t)/1 -> Sum/1
  phase/1 -> pi/180/1

== system umpc_wl_qp_beckymod2/signal generator/Drive_Signal/SignalForRamp_binary ==
  note: Should output 1 or -1,
      | so signal ramps UP to 1
      | or DOWN to 0.
  In1 : Inport
  Add : Sum  Inputs=+-
  Compare To Zero : simulink/Logic and Bit Operations/Compare To Zero  relop=>  OutDataTypeStr=uint8  ZeroCross=off
  Constant : Constant
  Data Type Conversion : DataTypeConversion  OutDataTypeStr=double
  Gain : Gain  Gain=2
  Out1 : Outport
  wires:
  In1/1 -> Compare To Zero/1
  Compare To Zero/1 -> Data Type Conversion/1
  Gain/1 -> Add/1
  Constant/1 -> Add/2
  Add/1 -> Out1/1
  Data Type Conversion/1 -> Gain/1

== system umpc_wl_qp_beckymod2/signal generator/Drive_Signal/SignalForSin_binary ==
  note: We want this to stay "high" for 1
      | second after the actual "enable"
      | is turned off...
  In1 : Inport
  Compare To Zero : simulink/Logic and Bit Operations/Compare To Zero  relop=>  OutDataTypeStr=uint8  ZeroCross=off
  Data Type Conversion : DataTypeConversion  OutDataTypeStr=double
  Out1 : Outport
  wires:
  In1/1 -> Compare To Zero/1
  Compare To Zero/1 -> Data Type Conversion/1
  Data Type Conversion/1 -> Out1/1

== system umpc_wl_qp_beckymod2/signal generator/Drive_Signal/Sinewave ==
  In2 : Inport
  2pi : Gain  Gain=2*pi
  first harmonic : Trigonometry  OutputSignalType=real
  integrate(omega*t) : DiscreteIntegrator  SampleTime=-1  ICPrevOutput=DiscIntNeverNeededParam  ICPrevScaledInput=DiscIntNeverNeededParam
  split cycle signal : Outport
  wires:
  In2/1 -> 2pi/1
  2pi/1 -> integrate(omega*t)/1
  integrate(omega*t)/1 -> first harmonic/1
  first harmonic/1 -> split cycle signal/1

== system umpc_wl_qp_beckymod2/signal generator/Drive_Signal1/AveragedAmp_filtered ==
  note: To avoid having signal "jump",
      | we want SMOOTH transitions
      | in frequency (i.e., a weighted sum
      | of current freq and freq some delta t ago)
  note: time constant 0.002sec
      | for 10kHz samping
  In1 : Inport
  Discrete Transfer Fcn : DiscreteTransferFcn  Numerator=[0.05]  Denominator=[1 -.95]
  Out1 : Outport
  wires:
  In1/1 -> Discrete Transfer Fcn/1
  Discrete Transfer Fcn/1 -> Out1/1

== system umpc_wl_qp_beckymod2/signal generator/Drive_Signal1/AveragedOffset_filtered ==
  note: To avoid having signal "jump",
      | we want SMOOTH transitions
      | in frequency (i.e., a weighted sum
      | of current freq and freq some delta t ago)
  note: c
  note: time constant 0.02sec
      | for 10kHz samping
  In1 : Inport
  Discrete Transfer Fcn : DiscreteTransferFcn  Numerator=[0.05]  Denominator=[1 -.95]
  Out1 : Outport
  wires:
  In1/1 -> Discrete Transfer Fcn/1
  Discrete Transfer Fcn/1 -> Out1/1

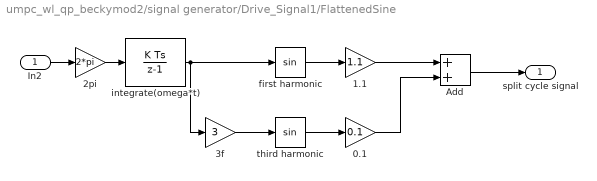
== system umpc_wl_qp_beckymod2/signal generator/Drive_Signal1/FlattenedSine ==
  In2 : Inport
  0.1 : Gain  Gain=0.1
  1.1 : Gain  Gain=1.1
  2pi : Gain  Gain=2*pi
  3f : Gain  Gain=3
  Add : Sum
  first harmonic : Trigonometry  OutputSignalType=real
  integrate(omega*t) : DiscreteIntegrator  SampleTime=-1  ICPrevOutput=DiscIntNeverNeededParam  ICPrevScaledInput=DiscIntNeverNeededParam
  third harmonic : Trigonometry  OutputSignalType=real
  split cycle signal : Outport
  wires:
  In2/1 -> 2pi/1
  2pi/1 -> integrate(omega*t)/1
  integrate(omega*t)/1 -> first harmonic/1, 3f/1
  3f/1 -> third harmonic/1
  first harmonic/1 -> 1.1/1
  third harmonic/1 -> 0.1/1
  1.1/1 -> Add/1
  0.1/1 -> Add/2
  Add/1 -> split cycle signal/1

== system umpc_wl_qp_beckymod2/signal generator/Drive_Signal1/SignalForRamp_binary ==
  note: Should output 1 or -1,
      | so signal ramps UP to 1
      | or DOWN to 0.
  In1 : Inport
  Add : Sum  Inputs=+-
  Compare To Zero : simulink/Logic and Bit Operations/Compare To Zero  relop=>  OutDataTypeStr=uint8  ZeroCross=off
  Constant : Constant
  Data Type Conversion : DataTypeConversion  OutDataTypeStr=double
  Gain : Gain  Gain=2
  Out1 : Outport
  wires:
  In1/1 -> Compare To Zero/1
  Compare To Zero/1 -> Data Type Conversion/1
  Gain/1 -> Add/1
  Constant/1 -> Add/2
  Add/1 -> Out1/1
  Data Type Conversion/1 -> Gain/1

== system umpc_wl_qp_beckymod2/signal generator/Drive_Signal1/SignalForSin_binary ==
  note: We want this to stay "high" for 1
      | second after the actual "enable"
      | is turned off...
  In1 : Inport
  Compare To Zero : simulink/Logic and Bit Operations/Compare To Zero  relop=>  OutDataTypeStr=uint8  ZeroCross=off
  Data Type Conversion : DataTypeConversion  OutDataTypeStr=double
  Out1 : Outport
  wires:
  In1/1 -> Compare To Zero/1
  Compare To Zero/1 -> Data Type Conversion/1
  Data Type Conversion/1 -> Out1/1

== system umpc_wl_qp_beckymod2/signal generator/Drive_Signal1/Sine Wave ==
  In2 : Inport
  2pi : Gain  Gain=2*pi
  first harmonic : Trigonometry  OutputSignalType=real
  integrate(omega*t) : DiscreteIntegrator  SampleTime=-1  ICPrevOutput=DiscIntNeverNeededParam  ICPrevScaledInput=DiscIntNeverNeededParam
  split cycle signal : Outport
  wires:
  In2/1 -> 2pi/1
  2pi/1 -> integrate(omega*t)/1
  integrate(omega*t)/1 -> first harmonic/1
  first harmonic/1 -> split cycle signal/1

== system umpc_wl_qp_beckymod2/signal generator/Drive_Signal2/AveragedAmp_filtered ==
  note: To avoid having signal "jump",
      | we want SMOOTH transitions
      | in frequency (i.e., a weighted sum
      | of current freq and freq some delta t ago)
  note: time constant 0.002sec
      | for 10kHz samping
  In1 : Inport
  Discrete Transfer Fcn : DiscreteTransferFcn  Numerator=[0.05]  Denominator=[1 -.95]
  Out1 : Outport
  wires:
  In1/1 -> Discrete Transfer Fcn/1
  Discrete Transfer Fcn/1 -> Out1/1

== system umpc_wl_qp_beckymod2/signal generator/Drive_Signal2/AveragedOffset_filtered ==
  note: To avoid having signal "jump",
      | we want SMOOTH transitions
      | in frequency (i.e., a weighted sum
      | of current freq and freq some delta t ago)
  note: c
  note: time constant 0.02sec
      | for 10kHz samping
  In1 : Inport
  Discrete Transfer Fcn : DiscreteTransferFcn  Numerator=[0.05]  Denominator=[1 -.95]
  Out1 : Outport
  wires:
  In1/1 -> Discrete Transfer Fcn/1
  Discrete Transfer Fcn/1 -> Out1/1

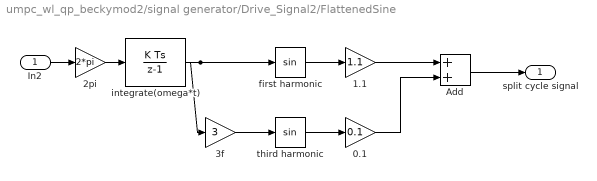
== system umpc_wl_qp_beckymod2/signal generator/Drive_Signal2/FlattenedSine ==
  In2 : Inport
  0.1 : Gain  Gain=0.1
  1.1 : Gain  Gain=1.1
  2pi : Gain  Gain=2*pi
  3f : Gain  Gain=3
  Add : Sum
  first harmonic : Trigonometry  OutputSignalType=real
  integrate(omega*t) : DiscreteIntegrator  SampleTime=-1  ICPrevOutput=DiscIntNeverNeededParam  ICPrevScaledInput=DiscIntNeverNeededParam
  third harmonic : Trigonometry  OutputSignalType=real
  split cycle signal : Outport
  wires:
  In2/1 -> 2pi/1
  2pi/1 -> integrate(omega*t)/1
  integrate(omega*t)/1 -> first harmonic/1, 3f/1
  3f/1 -> third harmonic/1
  first harmonic/1 -> 1.1/1
  third harmonic/1 -> 0.1/1
  1.1/1 -> Add/1
  0.1/1 -> Add/2
  Add/1 -> split cycle signal/1

== system umpc_wl_qp_beckymod2/signal generator/Drive_Signal2/SignalForRamp_binary ==
  note: Should output 1 or -1,
      | so signal ramps UP to 1
      | or DOWN to 0.
  In1 : Inport
  Add : Sum  Inputs=+-
  Compare To Zero : simulink/Logic and Bit Operations/Compare To Zero  relop=>  OutDataTypeStr=uint8  ZeroCross=off
  Constant : Constant
  Data Type Conversion : DataTypeConversion  OutDataTypeStr=double
  Gain : Gain  Gain=2
  Out1 : Outport
  wires:
  In1/1 -> Compare To Zero/1
  Compare To Zero/1 -> Data Type Conversion/1
  Gain/1 -> Add/1
  Constant/1 -> Add/2
  Add/1 -> Out1/1
  Data Type Conversion/1 -> Gain/1

== system umpc_wl_qp_beckymod2/signal generator/Drive_Signal2/SignalForSin_binary ==
  note: We want this to stay "high" for 1
      | second after the actual "enable"
      | is turned off...
  In1 : Inport
  Compare To Zero : simulink/Logic and Bit Operations/Compare To Zero  relop=>  OutDataTypeStr=uint8  ZeroCross=off
  Data Type Conversion : DataTypeConversion  OutDataTypeStr=double
  Out1 : Outport
  wires:
  In1/1 -> Compare To Zero/1
  Compare To Zero/1 -> Data Type Conversion/1
  Data Type Conversion/1 -> Out1/1

== system umpc_wl_qp_beckymod2/signal generator/Drive_Signal2/Sine Wave ==
  In2 : Inport
  2pi : Gain  Gain=2*pi
  first harmonic : Trigonometry  OutputSignalType=real
  integrate(omega*t) : DiscreteIntegrator  SampleTime=-1  ICPrevOutput=DiscIntNeverNeededParam  ICPrevScaledInput=DiscIntNeverNeededParam
  split cycle signal : Outport
  wires:
  In2/1 -> 2pi/1
  2pi/1 -> integrate(omega*t)/1
  integrate(omega*t)/1 -> first harmonic/1
  first harmonic/1 -> split cycle signal/1

== matlab function umpc_wl_qp_beckymod2/Hierarchical controller/Generate desired traj ==
function [pdes, dpdes, sdes, pdes_log] = desTraj(t, pos0, trajFreq, trajAmp)

omg = 2*pi*trajFreq;
pdes_log = double(pos0 + trajAmp*[0;-sin(omg*t);0]); % double
pdes = single(pdes_log);
dpdes = single(trajAmp*omg*[0;-cos(omg*t);0]);
sdes = single([0;0;1]);

== matlab function umpc_wl_qp_beckymod2/MATLAB Function ==
function freq = fcn(time, f_int, f_fin, T)
%#codegen

freq = f_int;
buffer_t = 0.0; %3.0
rel_time = time-buffer_t;
if rel_time > 0
    freq = f_int + (f_fin-f_int) * (rel_time/T);
end

if freq > f_fin
    freq = f_fin;
end

== matlab function umpc_wl_qp_beckymod2/Hierarchical controller/Convert inputs to single ==
function [ps, Rbs, dqs] = convertInp(p, Rb, dq)
% 
ps = single(p);
Rbs = single(Rb);
dqs = single(dq);

% Test noisy outputs
% dqs(1:3) = single(zeros(3,1));

== matlab function umpc_wl_qp_beckymod2/stateEst ==
function [p,Rb,dq,nmeas] = stateEst(t, qvicon, deadtime, lpfParams)
	% Low-pass filter
	% persistent Rbprev Rbdot eulprev v pprev tprevM
	persistent tprevP tprevM qvprev xhat Rbhat A Q R H P nmeas1 Rbvprev omgfilt lpfomg lpfR
	if isempty(tprevP)
		%fprintf(1, 'Initializing\n')
		tprevM = 0;
		tprevP = 0;
		qvprev = zeros(6,1);
		xhat = zeros(6,1); % positions
		Rbhat = eye(3);
		Rbvprev = eye(3);
		A = eye(6);
		Q = lpfParams(3) * diag([0.1 0.1 0.1 100 100 100]);
		R = lpfParams(4) * diag([0.1 0.1 0.1]);
		H = [eye(3) zeros(3,3)];
		P = eye(6);
		nmeas1 = 0;
		omgfilt = zeros(3,1);
		lpfomg = lpfParams(1);
		lpfR = lpfParams(2);
	end
	
% 	if t < deadtime
% 	if (qvicon(1) == 0)
% 		
% 		
% 	
% 	end
	
	% Prediction
	dt = t - tprevP;
	tprevP = t;
	A(1:3, 4:6) = dt * eye(3);
	xhat = A * xhat;
	P = A * P * A' + Q;
	% group
	Rbhat = Rbhat * expm(skew(omgfilt) * dt); % checked order; correct
	% not guaranteed SO(3) after this
	
	% Measurement if the vicon data changed
	if sum(isnan(qvicon)) == 0 && norm(qvicon - qvprev) > 1e-3
		nmeas1 = nmeas1 + 1;
		dt = t - tprevM;
		
		% Rbv = eul2rotm(qvicon(4:6)', 'ZYZ');
		Rbv = get_rotation_matrix(qvicon(4:6));
		
		if qvprev(1) ~= 0
			y = qvicon(1:3) - H * xhat;
			S = H * P * H' + R;
			K = P * H' / S;
			xhat = xhat + K * y;
			P = (eye(6) - K * H) * P;
			
			% Find Rbdot
			Rbdot = (Rbv - Rbvprev) / dt;
			% body-frame ang vel
			omgfilt = omgfilt + lpfomg * (unskew(Rbv' * Rbdot) - omgfilt);
% 			if (qvprev(1)==0) || (qvicon(1)==0)
% 				omgfilt = zeros(3,1);
% 			end

			% Correct orientation
			errHat = -Rbv' * Rbhat + Rbhat' * Rbv;
			Rbhat = Rbhat * expm(lpfR * errHat);
		end
		
		Rbvprev = Rbv;
		
		qvprev = qvicon;
		tprevM = t;
	end
	
	nmeas = nmeas1;
	% Outputs
	Rb = Rbhat;
	dq = [xhat(4:6); omgfilt];
	p = xhat(1:3);
end

function X = skew(v)
	X=[0   -v(3)  v(2);
	 v(3)    0  -v(1);
	-v(2)    v(1)   0  ];
end

function v = unskew(X)
	v = [X(3,2);X(1,3);X(2,1)];
end

== matlab function umpc_wl_qp_beckymod2/Hierarchical controller/Low-level control selector ==
% function [drv_amp, drv_pch, drv_roll, drv_bias, uquad_log, accdes_log] = convertU(uwlqp, uquad, accdes, useWL)
function [drv_amp, drv_pch, drv_roll, drv_bias, actualT0, ...
	uquad_log, accdes_log] = convertU(t, uquad, accdes, kquad, p, posdes, dq)

% use uquad
thrust = uquad(1);
momx = uquad(2);
momy = uquad(3);

% bias/initial lift to clear tether
Vmean = single(155);
udiff = single(-0.06);
uoffs = single(0);

if t > 0.1
	%Vmean = kquad(4) + kquad(1)*thrust;
	% stupid version PD for z
	Vmean = kquad(4) - clip(kquad(1)*(p(3)-posdes(3)) + kquad(5)*dq(3), -10, 10);
	
	% From static tests: drv_pch>0 => -momy, vR>vL (=>drv_roll<0) => -momx
	uoffs = uoffs - kquad(2)*momy;
	udiff = udiff + kquad(3)*momx;
end

% Clip and convert
vleft = clip(Vmean * (1 + udiff), 100, 170);
vright = clip(Vmean * (1 - udiff), 100, 170);
drv_pch = clip(double(Vmean * uoffs), -20, 20);

% This is same as target_driver_setup
drv_amp = double(abs((vleft-vright))/2+min(vleft,vright));
drv_roll = double((vleft-vright)/4 * 0.5);
drv_bias = double(max(vleft,vright)+2*abs(drv_pch)); % voltage

% Some function of Vmean
actualT0 = single(1);

% double for logging
uquad_log = double(uquad);
accdes_log = double(accdes);
end

== matlab function umpc_wl_qp_beckymod2/Phantom/start at three ==
function trigger = fcn(time)
%#codegen
trigger = 0;
if time > 0
   trigger = 1; 
end
if time > 0.1
   trigger = 0; 
end
